simulink model "ctyrkompart"  (Simulink 8.0)
settings: Solver=ode45  StartTime=0.0  StopTime=100  RelTol=1e-3
settings Model: Creator=polacmi1  LastModifiedBy=Jarda
settings DataIOCC: SignalLoggingSaveFormat=ModelDataLogs
settings DebuggingCC: FcnCallInpInsideContextMsg=EnableAllAsWarning

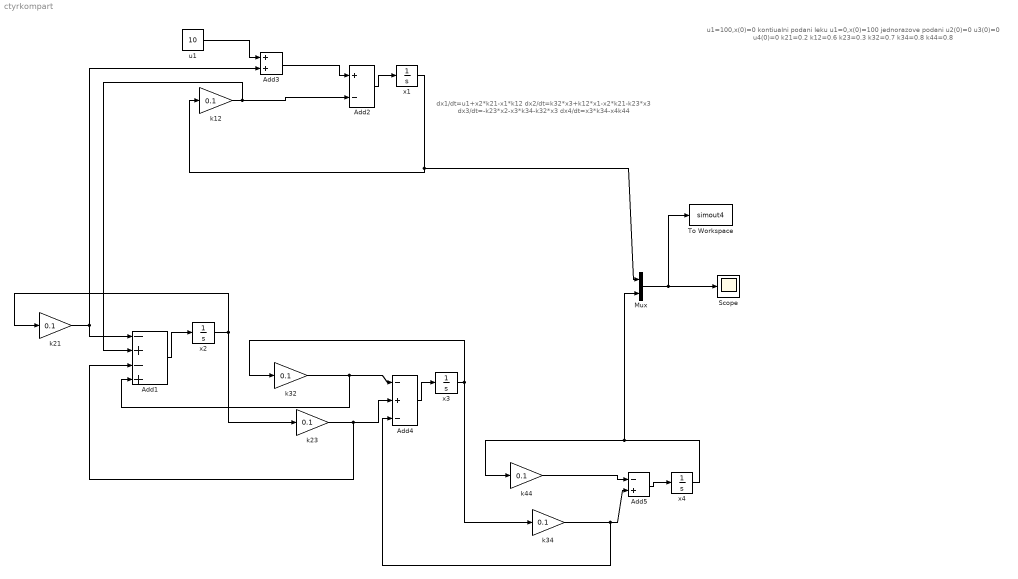
== system ctyrkompart ==
  note: u1=100,x(0)=0 kontiualni podani leku
      | u1=0,x(0)=100 jednorazove podani
      | u2(0)=0
      | u3(0)=0
      | u4(0)=0
      | k21=0.2
      | k12=0.6
      | k23=0.3
      | k32=0.7
      | k34=0.8
      | k44=0.8
  note: dx1/dt=u1+x2*k21-x1*k12
      |
      | dx2/dt=k32*x3+k12*x1-x2*k21-k23*x3
      |
      | dx3/dt=-k23*x2-x3*k34-k32*x3
      |
      | dx4/dt=x3*k34-x4k44
  Add1 : Sum  Inputs=-+-+
  Add2 : Sum  Inputs=+-
  Add3 : Sum
  Add4 : Sum  Inputs=-+-
  Add5 : Sum  Inputs=-+
  Mux : Mux  Inputs=2
  Scope : Scope
  To Workspace : ToWorkspace  VariableName=simout4  SampleTime=-1  SaveFormat=Timeseries
  k{12,21,23,32,34,44} (6 alike) : Gain  Gain=0.1
  u1 : Constant  Value=10
  x1 : Integrator  InitialCondition=100
  x2 : Integrator
  x3 : Integrator
  x4 : Integrator
  wires:
  x1/1 -> Mux/1, k12/1
  x2/1 -> k23/1, k21/1
  Add1/1 -> x2/1
  Add2/1 -> x1/1
  k12/1 -> Add2/2, Add1/2
  u1/1 -> Add3/1
  k21/1 -> Add3/2, Add1/1
  Add3/1 -> Add2/1
  Mux/1 -> To Workspace/1, Scope/1
  x3/1 -> k32/1, k34/1
  Add4/1 -> x3/1
  k32/1 -> Add4/1, Add1/4
  k23/1 -> Add4/2, Add1/3
  x4/1 -> k44/1, Mux/2
  Add5/1 -> x4/1
  k44/1 -> Add5/1
  k34/1 -> Add5/2, Add4/3
